simulink model "multibanddynamiccompression"  (R2014a)
settings: Solver=FixedStepDiscrete  StartTime=0.0  StopTime=Inf  RelTol=1e-3
InitFcn:
  | Ts = 1/44.1e3;
  | L = 8192;
values from neighbouring files (symbols this model uses):
  F = 75    [HelperAdaptiveNoiseCancellation.m]
libraries: dspindex x8, dspstat3 x2, dspvision x1, dspswit3 x1, dspsnks4 x1
CloseFcn:
  | clear Ts L
  | close all force
settings Model: Creator=The MathWorks Inc.
settings DebuggingCC: UnderspecifiedInitializationDetection=Classic

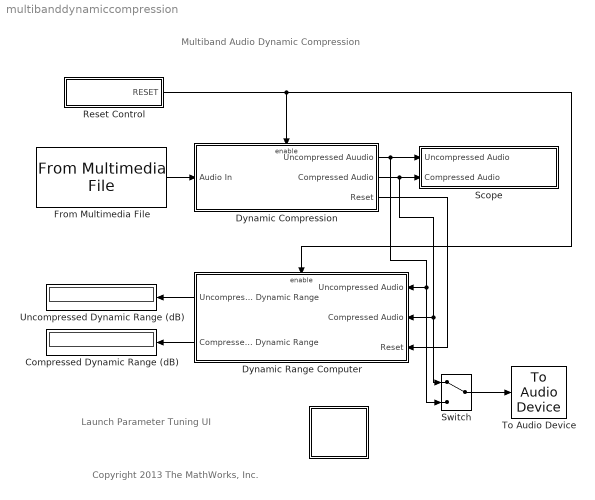
== system multibanddynamiccompression ==
  note: Copyright 2013 The MathWorks, Inc.
  note: Launch Parameter Tuning UI
  note: Multiband Audio Dynamic Compression
  " " : Subsystem  TreatAsAtomicUnit=on
      settings: OpenFcn=web(fullfile(matlabroot,'toolbox','dsp','dspdemos','html','audiomultibanddynamiccompressionexample.html'),'-helpbrowser')
      mask Display: disp('info')
  Compressed Dynamic Range (dB) : Display
  Dynamic Compression : Subsystem  TreatAsAtomicUnit=on
  Dynamic Range Computer : Subsystem  TreatAsAtomicUnit=on
  From Multimedia File : dspvision/From Multimedia File  inputFilename=guitar10min.ogg  loop=on  numPlays=inf  outputStreams=Audio only  videoDataType=single  audioDataType=double  inheritSampleTime=on  userDefinedSampleTime=1/30  noAudioOutput=off  isIntensityVideo=off  fourcc=RGB  colorVideoFormat=Separate color signals  outputEOF=off  dataOrg=Column-major  audioFrameSize=L  computeAudioFrameSize=off  outSamplingMode=Sample based
  Reset Control : Subsystem
  Scope : Subsystem  TreatAsAtomicUnit=on
  Switch : ManualSwitch
  To Audio Device : dspsnks4/To Audio Device  deviceName=Default  inheritSampleRate=on  sampleRate=44100  deviceDatatype=Determine from input data type  autoBufferSize=off  bufferSize=L  queueDuration=2.0  defaultOutputChannelMapping=on  outputChannelMapping=1:2
  Uncompressed Dynamic Range (dB) : Display
  wires:
  From Multimedia File/1 -> Dynamic Compression/1(Audio In)
  Reset Control/1(RESET) -> Dynamic Range Computer/Enable, Dynamic Compression/Enable
  Dynamic Compression/1("  Uncompressed Auudio") -> Scope/1(Uncompressed Audio), Switch/2, Dynamic Range Computer/1(Uncompressed Audio)
  Dynamic Compression/2("   Compressed Audio") -> Scope/2(Compressed Audio), Switch/1, Dynamic Range Computer/2(Compressed Audio)
  Switch/1 -> To Audio Device/1
  Dynamic Range Computer/1("   Uncompressed Dynamic Range") -> Uncompressed Dynamic Range (dB)/1
  Dynamic Range Computer/2("   Compressed Dynamic Range") -> Compressed Dynamic Range (dB)/1
  Dynamic Compression/3("  Reset") -> Dynamic Range Computer/3(" Reset")

== system multibanddynamiccompression/  ==

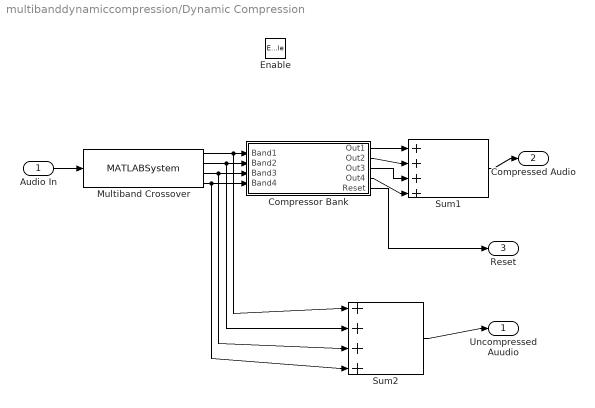
== system multibanddynamiccompression/Dynamic Compression ==
  Audio In : Inport
  Enable : EnablePort  StatesWhenEnabling=reset
  Compressor Bank : Subsystem  TreatAsAtomicUnit=on
  "Multiband Crossover  " : MATLABSystem  System=dspdemo.MultibandCrossoverFilter  SampleRate=44100  CrossoverFilterOrder=8  NumBands=4  CrossoverFrequencies=[120 1e3 3e3]
      mask Type: dspdemo.MultibandCrossoverFilter
      mask Display:
      | disp(['Multiband Crossover' char(10) 'Filter']);
      | port_label('input',1,'x');
  Sum1 : Sum  Inputs=|++++
  Sum2 : Sum  Inputs=|++++
  "  Uncompressed Auudio" : Outport
  "   Compressed Audio" : Outport  Port=2
  "  Reset" : Outport  Port=3
  wires:
  Audio In/1 -> "Multiband Crossover  "/1
  "Multiband Crossover  "/2 -> Sum2/2, Compressor Bank/2(Band2)
  "Multiband Crossover  "/3 -> Sum2/3, Compressor Bank/3(Band3)
  "Multiband Crossover  "/1 -> Sum2/1, Compressor Bank/1(Band1)
  "Multiband Crossover  "/4 -> Sum2/4, Compressor Bank/4(Band4)
  Sum2/1 -> "  Uncompressed Auudio"/1
  Sum1/1 -> "   Compressed Audio"/1
  Compressor Bank/1(Out1) -> Sum1/1
  Compressor Bank/2(Out2) -> Sum1/2
  Compressor Bank/3(Out3) -> Sum1/3
  Compressor Bank/4(Out4) -> Sum1/4
  Compressor Bank/5(Reset) -> "  Reset"/1

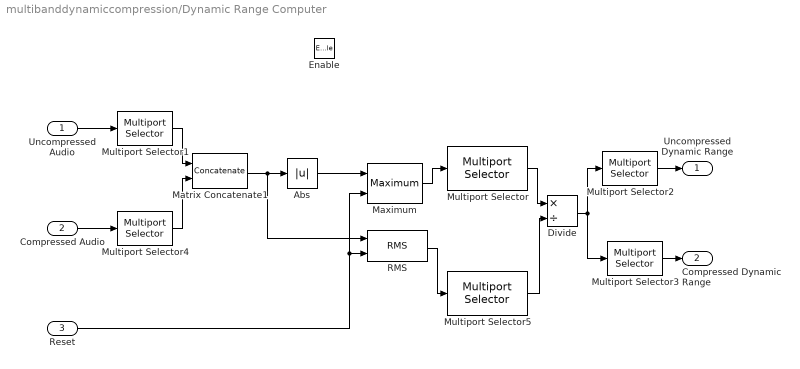
== system multibanddynamiccompression/Dynamic Range Computer ==
  Uncompressed Audio : Inport
  Compressed Audio : Inport  Port=2
  " Reset" : Inport  Port=3
  Enable : EnablePort  StatesWhenEnabling=reset
  Abs : Abs
  Divide : Product  Inputs=*/
  Matrix Concatenate1 : Concatenate  Mode=Multidimensional array  ConcatenateDimension=2
  Maximum : dspstat3/Maximum  fcn=Running  reset=Non-zero sample  InputProcessing=Columns as channels (frame based)  indexBase=One  operateOver=Each column  Dimension=1  colComp=on  operation=maximum  roiEnable=off  roiType=Rectangles  roiPortion=Entire ROI  roiOutput=Individual statistics for each ROI  roiFlag=off  accumDataTypeStr=Inherit: Same as product output  accumLastDataTypeStr=Inherit: Same as product output  roundingMode=Floor  overflowMode=off
  Multiport Selector : dspindex/Multiport Selector  rowsOrCols=Rows  idxCellArray={L}  idxErrMode=Clip Index
  Multiport Selector1 : dspindex/Multiport Selector  rowsOrCols=Columns  idxCellArray={1}  idxErrMode=Clip Index
  Multiport Selector2 : dspindex/Multiport Selector  rowsOrCols=Columns  idxCellArray={1}  idxErrMode=Clip Index
  Multiport Selector3 : dspindex/Multiport Selector  rowsOrCols=Columns  idxCellArray={2}  idxErrMode=Clip Index
  Multiport Selector4 : dspindex/Multiport Selector  rowsOrCols=Columns  idxCellArray={1}  idxErrMode=Clip Index
  Multiport Selector5 : dspindex/Multiport Selector  rowsOrCols=Rows  idxCellArray={L}  idxErrMode=Clip Index
  RMS : dspstat3/RMS  run=on  reset_popup=Non-zero sample  InputProcessing=Columns as channels (frame based)  directionMode=Each column  dimension=1  treatSBRowAsCol=on
  "   Uncompressed Dynamic Range" : Outport
  "   Compressed Dynamic Range" : Outport  Port=2
  wires:
  Uncompressed Audio/1 -> Multiport Selector1/1
  Compressed Audio/1 -> Multiport Selector4/1
  Multiport Selector1/1 -> Matrix Concatenate1/1
  Multiport Selector4/1 -> Matrix Concatenate1/2
  Matrix Concatenate1/1 -> Abs/1, RMS/1
  Multiport Selector2/1 -> "   Uncompressed Dynamic Range"/1
  Multiport Selector3/1 -> "   Compressed Dynamic Range"/1
  Abs/1 -> Maximum/1
  " Reset"/1 -> RMS/2, Maximum/2
  Maximum/1 -> Multiport Selector/1
  RMS/1 -> Multiport Selector5/1
  Multiport Selector/1 -> Divide/1
  Multiport Selector5/1 -> Divide/2
  Divide/1 -> Multiport Selector2/1, Multiport Selector3/1

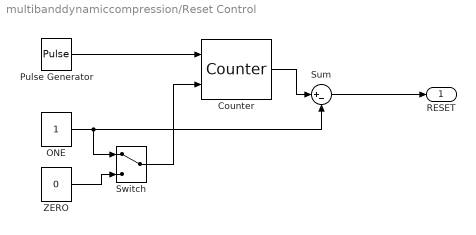
== system multibanddynamiccompression/Reset Control ==
  Counter : dspswit3/Counter  Direction=Up  CountEvent=Either edge  CounterSize=32 bits  MaxCount=1  InitialCount=0  Output=Count  HitValue=32  ResetInput=on  SamplesPerFrame=1  Ts=Ts * F  CntDtype=double  HitDtype=Logical
  ONE : Constant  VectorParams1D=off
  Pulse Generator : DiscretePulseGenerator  SampleTime=Ts * L
  Sum : Sum  Inputs=|+-
  Switch : ManualSwitch
  ZERO : Constant  Value=0  VectorParams1D=off
  RESET : Outport
  wires:
  ONE/1 -> Switch/1, Sum/2
  Switch/1 -> Counter/2
  Sum/1 -> RESET/1
  ZERO/1 -> Switch/2
  Pulse Generator/1 -> Counter/1
  Counter/1 -> Sum/1

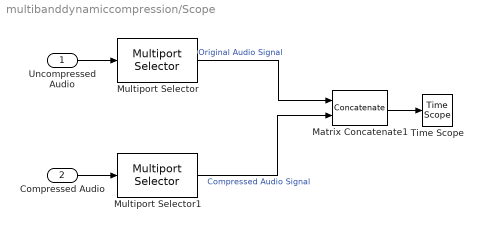
== system multibanddynamiccompression/Scope ==
  Uncompressed Audio : Inport
  Compressed Audio : Inport  Port=2
  Matrix Concatenate1 : Concatenate  Mode=Multidimensional array  ConcatenateDimension=2
  Multiport Selector : dspindex/Multiport Selector  rowsOrCols=Columns  idxCellArray={ 1 }  idxErrMode=Clip Index
  Multiport Selector1 : dspindex/Multiport Selector  rowsOrCols=Columns  idxCellArray={ 1 }  idxErrMode=Clip Index
  Time Scope : TimeScope  DefaultConfigurationName=spbscopes.TimeScopeBlockCfg
  wires:
  Multiport Selector/1 -> Matrix Concatenate1/1  "Original Audio Signal"
  Multiport Selector1/1 -> Matrix Concatenate1/2  "Compressed Audio Signal"
  Matrix Concatenate1/1 -> Time Scope/1
  Compressed Audio/1 -> Multiport Selector1/1
  Uncompressed Audio/1 -> Multiport Selector/1

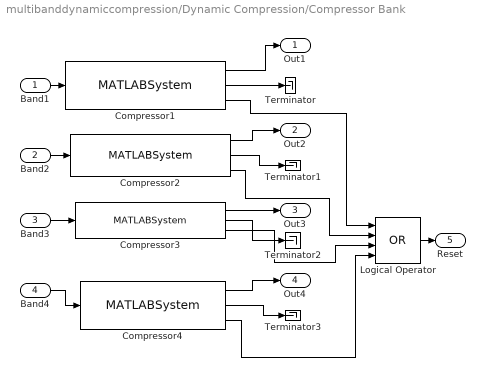
== system multibanddynamiccompression/Dynamic Compression/Compressor Bank ==
  Band1 : Inport
  Band2 : Inport  Port=2
  Band3 : Inport  Port=3
  Band4 : Inport  Port=4
  Compressor1 : MATLABSystem  System=dspdemo.DynamicRangeCompressor  SampleRate=44100  CompressionRatio=5  Threshold=-5  KneeWidth=5  AttackTime=5e-3  ReleaseTime=100e-3  MakeUpGain=0
      mask Type: dspdemo.DynamicRangeCompressor
      mask Display:
      | disp(['Dynamic Range' char(10) 'Compressor']);
      | port_label('input',1,'x');
      | port_label('output',1,'y');
      | port_label('output',2,'yLevel');
      | port_label('output',3,'propChanged');
  Compressor2 : MATLABSystem  System=dspdemo.DynamicRangeCompressor  SampleRate=44100  CompressionRatio=5  Threshold=-10  KneeWidth=5  AttackTime=5e-3  ReleaseTime=100e-3  MakeUpGain=0
      mask Type: dspdemo.DynamicRangeCompressor
      mask Display:
      | disp(['Dynamic Range' char(10) 'Compressor']);
      | port_label('input',1,'x');
      | port_label('output',1,'y');
      | port_label('output',2,'yLevel');
      | port_label('output',3,'propChanged');
  Compressor3 : MATLABSystem  System=dspdemo.DynamicRangeCompressor  SampleRate=44100  CompressionRatio=5  Threshold=-20  KneeWidth=5  AttackTime=2e-3  ReleaseTime=50e-3  MakeUpGain=0
      mask Type: dspdemo.DynamicRangeCompressor
      mask Display:
      | disp(['Dynamic Range' char(10) 'Compressor']);
      | port_label('input',1,'x');
      | port_label('output',1,'y');
      | port_label('output',2,'yLevel');
      | port_label('output',3,'propChanged');
  Compressor4 : MATLABSystem  System=dspdemo.DynamicRangeCompressor  SampleRate=44100  CompressionRatio=4  Threshold=-30  KneeWidth=5  AttackTime=2e-3  ReleaseTime=50e-3  MakeUpGain=0
      mask Type: dspdemo.DynamicRangeCompressor
      mask Display:
      | disp(['Dynamic Range' char(10) 'Compressor']);
      | port_label('input',1,'x');
      | port_label('output',1,'y');
      | port_label('output',2,'yLevel');
      | port_label('output',3,'propChanged');
  Logical Operator : Logic  Operator=OR  Inputs=4  AllPortsSameDT=off  OutDataTypeStr=boolean
  Terminator{,1..3} (4 alike) : Terminator
  Out1 : Outport
  Out2 : Outport  Port=2
  Out3 : Outport  Port=3
  Out4 : Outport  Port=4
  Reset : Outport  Port=5
  wires:
  Band1/1 -> Compressor1/1
  Band2/1 -> Compressor2/1
  Band3/1 -> Compressor3/1
  Band4/1 -> Compressor4/1
  Compressor1/1 -> Out1/1
  Compressor2/1 -> Out2/1
  Compressor3/1 -> Out3/1
  Compressor4/1 -> Out4/1
  Logical Operator/1 -> Reset/1
  Compressor1/2 -> Terminator/1
  Compressor2/2 -> Terminator1/1
  Compressor3/2 -> Terminator2/1
  Compressor4/2 -> Terminator3/1
  Compressor1/3 -> Logical Operator/1
  Compressor2/3 -> Logical Operator/2
  Compressor3/3 -> Logical Operator/3
  Compressor4/3 -> Logical Operator/4
